simulink model "cv_model_CMORPH_5M"  (R2024a)
settings: Solver=ode23t  StartTime=0  StopTime=1431  FixedStep=0.0005  MaxStep=.01  RelTol=1e-4
model workspace (MAT data in the model file):
  test = 0
undefined symbols (not defined in the file): A_cheb_09_1, B_cheb_09_1, C_cheb_09_1
libraries: simulink_extras x2, SignalEditorBlockLib x1
(part 2 of 3)

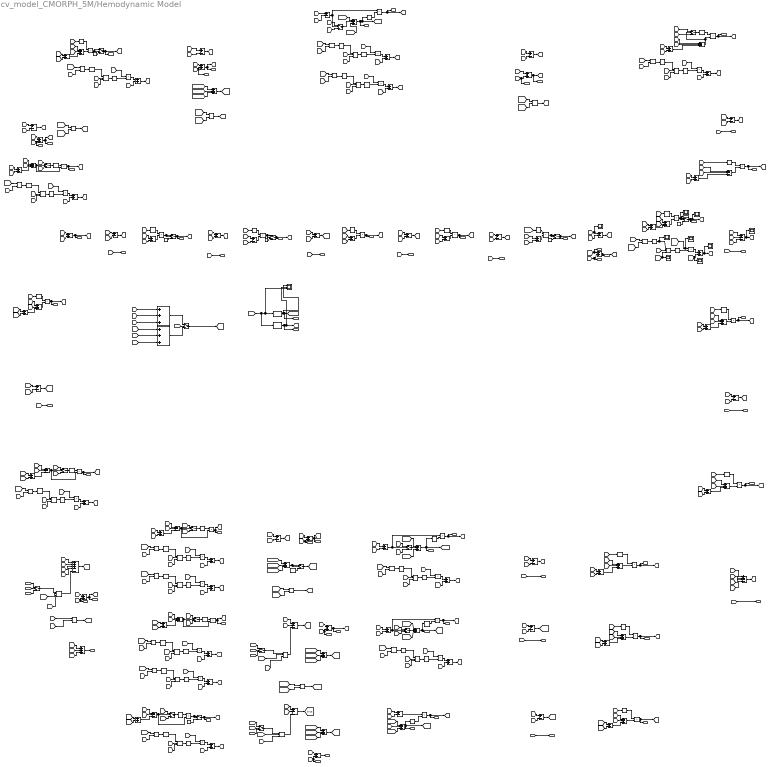
== system cv_model_CMORPH_5M/Hemodynamic Model ==
  note: Zero Pressure Volume
  note: Zero Pressure Volume
  note: Zero Pressure Volume
  note: Reduced Compliance at Negative Pressure
  note: Reduced Compliance at Negative Pressure
  note: Zero Pressure Volume
  note: Total Volume
  note: Zero Pressure Volume
  note: Update Zero Pressure Volume from Reflex
  note: Zero Pressure Volume
  note: Update Zero Pressure Volume from Reflex
  note: Zero Pressure Volume
  note: Zero Pressure Volume
  note: Zero Pressure Volume
  note: Zero Pressure Volume
  note: Zero Pressure Volume
  note: Total Volume
  note: Update Zero Pressure Volume from Reflex
  note: Total Volume
  note: Flow into Right Atrium
  note: Flow into Compartment 14
  note: Flow Out of Compartment 9
  note: Total Volume
  note: Vessel Collapse Before
  note: Vessel Collapse After
  note: Flow Out of Compartment 11
  note: Total Volume
  note: Flow Out of Compartment 13
  note: Vessel Collapse
  note: Lower Body Microvascular Resistance
  note: Flow into Compartment 12
  note: Splanchnic Circulation Microvascular Resistance
  note: Vessel Collapse
  note: Flow into Compartment 10
  note: Renal Circulation Microvascular Resistance
  note: Vessel Collapse
  note: Flow into Compartment 8
  note: 2: Brachiocephalic Arteries
  note: Flow into Compartment 7
  note: Upper Body Microvascular Resistance
  note: Vessel Collapse After
  note: Flow into Compartment 3
  note: Vessel Collapse Model
  note: Flow into Compartment 2
  note: Vessel Collapse Before
  note: Flow into Compartment 6
  note: 3: Upper Body Arteries
  note: 6: Thoracic Aorta
  note: 7: Abdominal Aorta
  note: 8: Renal Arteries
  note: 9: Renal Veins
  note: 10: Splanchnic Arteries
  note: 11: Splanchnic Veins
  note: 12: Lower Body Arteries
  note: 13: Lower Body Veins
  note: Vessel Collapse Before
  note: Vessel Collapse After
  note: 14: Abdominal Veins
  note: Flow into Compartment 15
  note: Total Volume
  note: Vessel Collapse
  note: 15: Thoracic IVC
  note: Flow Out of Compartment 15
  note: 4: Upper Body Veins
  note: Vessel Collapse
  note: Flow into Compartment 5
  note: 5: SVC
  note: 1: Ascending Aorta
  note: Vessel Collapse
  note: Total Volume
  note: Flow Out of Compartment 5
  note: Right Atrium
  note: Flow into Right Ventricle
  note: Right Ventricle
  note: Flow into Pulmonary Arteries
  note: Pulmonary Arteries
  note: Pulmonary Microvascular Resistance
  note: Pulmonary Veins
  note: Flow Out of Pulmonary Veins
  note: Left Atrium
  note: Flow into Left Ventricle
  note: Left Ventricle
  note: Flow Out of Left Ventricle
  note: Vessel Collapse
  note: Total Volume
  note: Total Hydrostatic Pressure into lower venous system for interstitial flow division
  note: Interstitial Flow to Splanchnic Veins
  note: Interstitial Flow to Lower Body Veins
  note: Interstitial Flow to Abdominal Veins
  note: Transfer Function for Vint
  note: Transfer Function for Qint
  note: Flow and Volume to Interstitial Space
  note: Reduced Compliance at Negative Pressure
  note: Reduced Compliance at Negative Pressure
  note: Reduced Compliance at Negative Pressure
  note: Reduced Compliance at Negative Pressure
  note: Zero Pressure Volume
  note: Zero Pressure Volume
  note: Update Zero Pressure Volume from Reflex
  Constant{1..6} (6 alike) : Constant  Value=0
  Math Function{,1,4,9..12,15..16,19..21,24,29,34,37..38,41,44..49} (24 alike) : Math  Operator=reciprocal  SignedPower=on
  Math Function{2,5,7,13,17,22,25..26,30..31,35,39,42,50} (14 alike) : Math  SignedPower=on
  Math Function{3,6,8,14,18,23,27..28,32..33,36,40,43,51} (14 alike) : Math  Operator=log  SignedPower=on
  Product{,1,4,7,10..11,14..15,18..19,22,25,28,31,34,37,40,43} (18 alike) : Product  InputSameDT=on  SaturateOnIntegerOverflow=on  OutDataTypeStr=Inherit: Same as first input
  Product{2,5,8,12,16,20,23,26,29,32,35,38,41,44} (14 alike) : Product  Inputs=*/  InputSameDT=on  SaturateOnIntegerOverflow=on  OutDataTypeStr=Inherit: Same as first input
  Product{3,6,9,13,17,21,24,27,30,33,36,39,42,45} (14 alike) : Product  Inputs=**/  InputSameDT=on  SaturateOnIntegerOverflow=on  OutDataTypeStr=Inherit: Same as first input
  Scope : Scope  NumInputPorts=3
  Scope{1..9} (9 alike) : Scope
  Sum{,3,12,16,20,44..48,52,55..68} (25 alike) : Sum  Inputs=+-  InputSameDT=on  SaturateOnIntegerOverflow=on  OutDataTypeStr=Inherit: Same as first input
  Sum{1..2,21,23,28,33,36,49,54,70..71} (11 alike) : Sum  Inputs=+--  InputSameDT=on  SaturateOnIntegerOverflow=on  OutDataTypeStr=Inherit: Same as first input
  Sum{9..11,13,17,37,40} (7 alike) : Sum  Inputs=+-+  InputSameDT=on  SaturateOnIntegerOverflow=on  OutDataTypeStr=Inherit: Same as first input
  Sum{4..6,8,14,18,24..27,29..31,34..35,38..39,41..43,50..51,77..92} (38 alike) : Sum  InputSameDT=on  SaturateOnIntegerOverflow=on  OutDataTypeStr=Inherit: Same as first input
  Sum{7,15,19,22,32,69,73..76,93} (11 alike) : Sum  Inputs=+++  InputSameDT=on  SaturateOnIntegerOverflow=on  OutDataTypeStr=Inherit: Same as first input
  Sum53 : Sum  Inputs=+---  InputSameDT=on  SaturateOnIntegerOverflow=on  OutDataTypeStr=Inherit: Same as first input
  Sum72 : Sum  Inputs=+++--  InputSameDT=on  SaturateOnIntegerOverflow=on  OutDataTypeStr=Inherit: Same as first input
  Switch{1..14,21} (15 alike) : Switch
  Switch{16,18..20} (4 alike) : Switch  Threshold=0.5
  Switch17 : Switch  Criteria=u2 > Threshold  Threshold=5
  Transfer Fcn (with initial states) : simulink_extras/Additional Linear/Transfer Fcn (with initial states)  N=[1 0]  D=[276 1]  X0=0
  Transfer Fcn (with initial states)1 : simulink_extras/Additional Linear/Transfer Fcn (with initial states)  N=[1]  D=[276 1]  X0=0
  ZV1 : Constant  Value=5
  kool{1..20} (20 alike) : Product  Inputs=**  InputSameDT=on  SaturateOnIntegerOverflow=on  OutDataTypeStr=Inherit: Same as first input
  kool21 : Product  Inputs=*/*  InputSameDT=on  SaturateOnIntegerOverflow=on  OutDataTypeStr=Inherit: Same as first input
  kool22 : Product  Inputs=*/*  InputSameDT=on  SaturateOnIntegerOverflow=on  OutDataTypeStr=Inherit: Same as first input
  kool23 : Product  Inputs=*/*  InputSameDT=on  SaturateOnIntegerOverflow=on  OutDataTypeStr=Inherit: Same as first input
  kool{24..29} (6 alike) : Product  Inputs=*/  InputSameDT=on  SaturateOnIntegerOverflow=on  OutDataTypeStr=Inherit: Same as first input
  Qlo : Outport
  Q2i : Outport  Port=2
  Q3i : Outport  Port=3
  Q4i : Outport  Port=4
  Q5i : Outport  Port=5
  Q5o : Outport  Port=6
  Q6i : Outport  Port=7
  Q7i : Outport  Port=8
  Q8i : Outport  Port=9
  Q9i : Outport  Port=10
  Q9o : Outport  Port=11
  Q10i : Outport  Port=12
  Q11i : Outport  Port=13
  Q11o : Outport  Port=14
  Q12i : Outport  Port=15
  Q13i : Outport  Port=16
  Q13o : Outport  Port=17
  Q14i : Outport  Port=18
  Q15i : Outport  Port=19
  Q15o : Outport  Port=20
  Qrai : Outport  Port=21
  Qri : Outport  Port=22
  Qro : Outport  Port=23
  Qpv : Outport  Port=24
  Qlai : Outport  Port=25
  Qli : Outport  Port=26
  Qint : Outport  Port=27
  Vint : Outport  Port=28
  RubNew : Outport  Port=29
  RrcNew : Outport  Port=30
  RscNew : Outport  Port=31
  RlcNew : Outport  Port=32
  zv1 : Outport  Port=33
  zv2 : Outport  Port=34
  zv3 : Outport  Port=35
  zv4 : Outport  Port=36
  zv5 : Outport  Port=37
  zv6 : Outport  Port=38
  zv7 : Outport  Port=39
  zv8 : Outport  Port=40
  zv9 : Outport  Port=41
  zv10 : Outport  Port=42
  zv11 : Outport  Port=43
  zv12 : Outport  Port=44
  zv13 : Outport  Port=45
  zv14 : Outport  Port=46
  zv15 : Outport  Port=47
  zvra : Outport  Port=48
  zvrv : Outport  Port=49
  zvpa : Outport  Port=50
  zvpv : Outport  Port=51
  zvla : Outport  Port=52
  zvlv : Outport  Port=53
  V3a : Outport  Port=54
  V4a : Outport  Port=55
  V5a : Outport  Port=56
  V9a : Outport  Port=57
  V11a : Outport  Port=58
  V13a : Outport  Port=59
  V14a : Outport  Port=60
  Vlva : Outport  Port=61
  Vl_dist : Outport  Port=62
  Qlo1 : Outport  Port=63
  tag scope: C11neg=global, C14neg=global, C3neg=global, C4neg=global, C5neg=global, C9neg=global, Q10i=global, Q11i=global, Q11o=global, Q12i=global, Q13i=global, Q13o=global, Q15i=global, Q15o=global, Q2i=global, Q3i=global, Q4i=global, Q5i=global, Q5o=global, Q6i=global, Q7i=global, Q8i=global, Q9i=global, Q9o=global, Qint=global, Qlai=global, Qli=global, Qlo=global, Qpv=global, Qrai=global, Qri=global, Qro=global, R11a=global, R11b=global, R13b=global, R14a=global, R1a=global, R3b=global, R4a=global, R5a=global, R9a=global, R9b=global, RlcNew=global, RrcNew=global, Rrcb=global, RscNew=global, Rscb=global, RubNew=global, Ruba=global, Rubb=global, V11a=global, V14a=global, V3a=global, V4a=global, V5a=global, V9a=global, Vint=global, Vl=global, ZV11=global, ZV13=global, ZV4=global, ZV9=global, dV10=global, dV11=global, dV12=global, dV13=global, dV14=global, dV15=global, dV1=global, dV2=global, dV3=global, dV4=global, dV5=global, dV6=global, dV7=global, dV8=global, dV9=global, dVl=global, dVla=global, dVpa=global, dVpv=global, dVr=global, dVra=global, hTotal=global
  wires:
  [P1] -> Sum1/1
  Sum1/1 -> kool4/2
  kool4/1 -> Q2i/1, [Q2i]
  Math Function/1 -> kool4/1
  [R2] -> Math Function/1
  [P2] -> Sum1/2
  Sum78/1 -> Sum1/3
  [R3b] -> Switch3/3
  Sum4/1 -> [R3b]
  [P3] -> Sum2/2
  [ZV3] -> Product3/3
  [P2] -> Sum2/1
  Math Function2/1 -> Product1/2
  Math Function3/1 -> Product3/1
  Product1/1 -> Sum4/1
  [V3a] -> Product3/2
  Product2/1 -> Math Function3/1
  [Rhigh] -> Product1/1
  Sum2/1 -> kool1/2, Switch3/2
  kool1/1 -> [Q3i], Q3i/1
  [R3] -> Switch3/1
  Product3/1 -> Math Function2/1
  [epsilon] -> Product2/1
  Sum79/1 -> Sum2/3
  Math Function1/1 -> kool1/1
  Switch3/1 -> Math Function1/1
  [R3] -> Sum4/2
  [Rhigh] -> Product2/2
  Sum8/1 -> [Rubb]
  Math Function4/1 -> Product/2
  Math Function7/1 -> Product7/2
  Product8/1 -> Math Function8/1
  Product9/1 -> Math Function7/1
  Math Function6/1 -> Product6/1
  [V4a] -> Product9/2
  [ZV3] -> Product6/3
  [P4] -> Sum3/2
  Product7/1 -> Sum8/1
  Product4/1 -> Sum6/1
  Sum3/1 -> Product/1, Switch1/2
  [epsilon] -> Product8/1
  [ZV4] -> Product9/3
  [Rhigh] -> Product7/1
  [Rub] -> Sum8/2
  Math Function8/1 -> Product9/1
  [Rhigh] -> Product5/2
  [Rhigh] -> Product8/2
  [rupdelt] -> Sum7/1
  Math Function5/1 -> Product4/2
  Sum5/1 -> [V3a], V3a/1
  [Rubb] -> Switch1/3
  Product5/1 -> Math Function6/1
  [ZV3] -> zv3/1, Sum5/2
  [Ruba] -> Switch1/1
  [V3] -> Sum5/1
  [V3a] -> Product6/2
  Product6/1 -> Math Function5/1
  [epsilon] -> Product5/1
  Switch1/1 -> Sum7/2
  [Rub] -> Sum6/2
  [rupdeltCP] -> Sum7/3
  Sum6/1 -> [Ruba]
  [Rhigh] -> Product4/1
  Sum7/1 -> [RubNew], Math Function4/1, RubNew/1
  [P3] -> Sum3/1
  Product/1 -> [Q4i], Q4i/1
  [P6] -> Sum9/2
  [P1] -> Sum9/1
  [R6] -> Math Function9/1
  Sum82/1 -> Sum9/3
  Sum9/1 -> kool2/2
  kool2/1 -> [Q6i], Q6i/1
  Math Function9/1 -> kool2/1
  Sum83/1 -> Sum10/3
  Math Function10/1 -> kool3/1
  kool3/1 -> [Q7i], Q7i/1
  [R7] -> Math Function10/1
  Sum10/1 -> kool3/2
  [P7] -> Sum10/2
  [P6] -> Sum10/1
  [P8] -> Sum11/2
  [R8] -> Math Function11/1
  Sum11/1 -> kool5/2
  [P7] -> Sum11/1
  Sum85/1 -> Sum11/3
  kool5/1 -> [Q8i], Q8i/1
  Math Function11/1 -> kool5/1
  [Rrcb] -> Switch2/3
  [Rhigh] -> Product11/1
  Sum14/1 -> [Rrcb]
  Product10/1 -> Q9i/1, [Q9i]
  Math Function13/1 -> Product11/2
  Switch2/1 -> Sum15/2
  [P9] -> Sum12/2
  [epsilon] -> Product12/1
  [V9a] -> Product13/2
  Product13/1 -> Math Function13/1
  Math Function12/1 -> Product10/2
  [P8] -> Sum12/1
  [Rhigh] -> Product12/2
  Product12/1 -> Math Function14/1
  [rkdeltCP] -> Sum15/3
  [ZV9] -> Product13/3
  Product11/1 -> Sum14/1
  [Rrc] -> Switch2/1
  [Rrc] -> Sum14/2
  Sum12/1 -> Product10/1, Switch2/2
  [rkdelt] -> Sum15/1
  Sum15/1 -> RrcNew/1, [RrcNew], Math Function12/1
  Math Function14/1 -> Product13/1
  [P10] -> Sum13/2
  [R10] -> Math Function15/1
  Math Function15/1 -> kool6/1
  Sum87/1 -> Sum13/3
  kool6/1 -> [Q10i], Q10i/1
  [P7] -> Sum13/1
  Sum13/1 -> kool6/2
  [Rscb] -> Switch4/3
  [P11] -> Sum16/2
  [ZV11] -> Product17/3
  [epsilon] -> Product16/1
  Math Function17/1 -> Product15/2
  [Rsc] -> Switch4/1
  Product15/1 -> Sum18/1
  [rspdelt] -> Sum19/1
  Product16/1 -> Math Function18/1
  Math Function18/1 -> Product17/1
  Product17/1 -> Math Function17/1
  [V11a] -> Product17/2
  [rspdeltCP] -> Sum19/3
  Switch4/1 -> Sum19/2
  [Rhigh] -> Product16/2
  Sum18/1 -> [Rscb]
  [Rhigh] -> Product15/1
  Math Function16/1 -> Product14/2
  Sum16/1 -> Product14/1, Switch4/2
  Sum19/1 -> [RscNew], Math Function16/1, RscNew/1
  Product14/1 -> Q11i/1, [Q11i]
  [P10] -> Sum16/1
  [Rsc] -> Sum18/2
  [P12] -> Sum17/2
  Sum89/1 -> Sum17/3
  Math Function19/1 -> kool7/1
  Sum17/1 -> kool7/2
  [R12] -> Math Function19/1
  [P7] -> Sum17/1
  kool7/1 -> [Q12i], Q12i/1
  Math Function20/1 -> Product18/2
  Sum22/1 -> [RlcNew], Math Function20/1, RlcNew/1
  [rlldeltCP] -> Sum22/3
  [Rlc] -> Sum22/2
  Product18/1 -> Q13i/1, [Q13i]
  [rlldelt] -> Sum22/1
  [P13] -> Sum20/2
  Sum20/1 -> Product18/1
  [P12] -> Sum20/1
  [R13] -> Sum24/2
  [R13] -> Switch6/1
  [R13b] -> Switch6/3
  Sum24/1 -> [R13b]
  Product19/1 -> Sum24/1
  [Rhigh] -> Product19/1
  Product20/1 -> Math Function23/1
  [Rhigh] -> Product20/2
  Math Function22/1 -> Product19/2
  Math Function23/1 -> Product21/1
  Constant1/1 -> Switch5/3
  [V14a] -> Product21/2
  [epsilon] -> Product20/1
  [ZV14] -> Product21/3
  kool8/1 -> Switch5/2, Switch5/1
  [P14] -> Sum21/2
  Switch5/1 -> [Q13o], Q13o/1
  Switch6/1 -> Math Function21/1
  Sum21/1 -> kool8/2, Switch6/2
  Sum90/1 -> Sum21/3
  Product21/1 -> Math Function22/1
  Math Function21/1 -> kool8/1
  [P13] -> Sum21/1
  [R11] -> Sum27/2
  [epsilon] -> Product26/1
  Product26/1 -> Math Function28/1
  Math Function25/1 -> Product25/2
  kool9/1 -> Q11o/1, [Q11o]
  [ZV14] -> Product27/3
  Product23/1 -> Math Function27/1
  Product27/1 -> Math Function25/1
  Math Function27/1 -> Product24/1
  [epsilon] -> Product23/1
  [V11] -> Sum26/1
  Math Function28/1 -> Product27/1
  [R11] -> Sum25/2
  [V14a] -> Product27/2
  [Rhigh] -> Product25/1
  Switch7/1 -> Math Function24/1
  [Rhigh] -> Product22/1
  [Rhigh] -> Product23/2
  Product24/1 -> Math Function26/1
  Product25/1 -> Sum25/1
  Product22/1 -> Sum27/1
  Sum25/1 -> [R11b]
  [P11] -> Sum23/1
  Sum23/1 -> Switch7/2, kool9/2
  Sum26/1 -> [V11a], V11a/1
  [R11a] -> Switch7/1
  Math Function26/1 -> Product22/2
  [ZV11] -> Product24/3
  [P14] -> Sum23/2
  [ZV11] -> zv11/1, Sum26/2
  Math Function24/1 -> kool9/1
  [R11b] -> Switch7/3
  [Rhigh] -> Product26/2
  [V11a] -> Product24/2
  Sum27/1 -> [R11a]
  Sum88/1 -> Sum23/3
  [Rhigh] -> Product31/1
  [R9] -> Sum29/2
  [V14a] -> Product33/2
  Switch8/1 -> Math Function29/1
  Product31/1 -> Sum29/1
  Math Function33/1 -> Product33/1
  Math Function32/1 -> Product30/1
  [Rhigh] -> Product32/2
  kool10/1 -> Q9o/1, [Q9o]
  [V9] -> Sum30/1
  Math Function30/1 -> Product31/2
  [epsilon] -> Product29/1
  [P14] -> Sum28/2
  [ZV9] -> zv9/1, Sum30/2
  [Rhigh] -> Product28/1
  Sum30/1 -> [V9a], V9a/1
  [Rhigh] -> Product29/2
  Math Function29/1 -> kool10/1
  [ZV14] -> Product33/3
  [P9] -> Sum28/1
  [epsilon] -> Product32/1
  Sum86/1 -> Sum28/3
  [R9a] -> Switch8/1
  Product29/1 -> Math Function32/1
  Product28/1 -> Sum31/1
  [R9b] -> Switch8/3
  Sum31/1 -> [R9a]
  [R9] -> Sum31/2
  Product32/1 -> Math Function33/1
  Math Function31/1 -> Product28/2
  [ZV9] -> Product30/3
  Sum28/1 -> kool10/2, Switch8/2
  Product33/1 -> Math Function30/1
  Product30/1 -> Math Function31/1
  [V9a] -> Product30/2
  Sum29/1 -> [R9b]
  [Q13o] -> Sum32/3
  Sum32/1 -> Q14i/1
  [Q11o] -> Sum32/2
  [Q9o] -> Sum32/1
  Math Function36/1 -> Product36/1
  [R14] -> Switch9/3
  [R14a] -> Switch9/1
  Switch9/1 -> Math Function34/1
  [ZV14] -> Sum34/2, zv14/1
  Sum35/1 -> [R14a]
  Math Function35/1 -> Product34/2
  [P15] -> Sum33/2
  [Rhigh] -> Product34/1
  [V14] -> Sum34/1
  [V14a] -> Product36/2
  Product35/1 -> Math Function36/1
  [R14] -> Sum35/2
  Sum91/1 -> Sum33/3
  [ZV14] -> Product36/3
  [Rhigh] -> Product35/2
  Product36/1 -> Math Function35/1
  kool11/1 -> Q15i/1, [Q15i]
  Math Function34/1 -> kool11/1
  [P14] -> Sum33/1
  Sum33/1 -> Switch9/2, kool11/2
  [epsilon] -> Product35/1
  Sum34/1 -> V14a/1, [V14a]
  Product34/1 -> Sum35/1
  Sum92/1 -> Sum36/3
  [R15] -> Math Function37/1
  [P15] -> Sum36/1
  Sum36/1 -> kool12/2
  kool12/1 -> Q15o/1, [Q15o]
  [Pra] -> Sum36/2
  Math Function37/1 -> kool12/1
  [V4a] -> Product39/2
  Sum39/1 -> [R4a]
  Math Function39/1 -> Product37/2
  Product37/1 -> Sum39/1
  [Rhigh] -> Product37/1
  [R4] -> Sum39/2
  Product39/1 -> Math Function39/1
  [P5] -> Sum37/2
  [Rhigh] -> Product38/2
  Product38/1 -> Math Function40/1
  Math Function40/1 -> Product39/1
  [V4] -> Sum38/1
  Switch10/1 -> Q5i/1, [Q5i]
  [ZV4] -> Product39/3
  kool13/1 -> Switch10/2, Switch10/1
  Sum80/1 -> Sum37/3
  Math Function38/1 -> kool13/1
  [P4] -> Sum37/1
  Sum37/1 -> kool13/2
  [R4a] -> Math Function38/1
  Constant2/1 -> Switch10/3
  [epsilon] -> Product38/1
  Sum38/1 -> V4a/1, [V4a]
  Math Function42/1 -> Product40/2
  kool14/1 -> Q5o/1, [Q5o]
  [ZV5] -> zv5/1, Sum41/2
  Sum41/1 -> V5a/1, [V5a]
  [epsilon] -> Product41/1
  Math Function41/1 -> kool14/1
  [Rhigh] -> Product40/1
  Sum40/1 -> kool14/2, Switch11/2
  [P5] -> Sum40/1
  Math Function43/1 -> Product42/1
  [R5a] -> Switch11/1
  [ZV5] -> Product42/3
  [Pra] -> Sum40/2
  [R5] -> Sum42/2
  Product40/1 -> Sum42/1
  [V5] -> Sum41/1
  [Rhigh] -> Product41/2
  [V5a] -> Product42/2
  Product42/1 -> Math Function42/1
  Switch11/1 -> Math Function41/1
  [R5] -> Switch11/3
  Sum42/1 -> [R5a]
  Product41/1 -> Math Function43/1
  Sum81/1 -> Sum40/3
  [Q15o] -> Sum43/2
  [Q5o] -> Sum43/1
  Sum43/1 -> Qrai/1, [Qrai]
  [R_tri] -> Math Function44/1
  Sum44/1 -> kool15/2
  kool15/1 -> Switch12/1, Switch12/2
  Math Function44/1 -> kool15/1
  Constant3/1 -> Switch12/3
  [Pra] -> Sum44/1
  [Pr] -> Sum44/2
  Switch12/1 -> Qri/1, [Qri]
  [Ppa] -> Sum45/2
  kool16/1 -> Switch13/2, Switch13/1
  [Rpa] -> Math Function45/1
  Math Function45/1 -> kool16/1
  Constant4/1 -> Switch13/3
  Sum45/1 -> kool16/2
  Switch13/1 -> [Qro], Qro/1
  [Pr] -> Sum45/1
  [Ppv] -> Sum46/2
  [Ppa] -> Sum46/1
  kool17/1 -> [Qpv], Qpv/1
  Sum46/1 -> kool17/2
  [Rpc] -> Math Function46/1
  Math Function46/1 -> kool17/1
  [Rpv] -> Math Function47/1
  Sum47/1 -> kool18/2
  kool18/1 -> [Qlai], Qlai/1
  Math Function47/1 -> kool18/1
  [Ppv] -> Sum47/1
  [Pla] -> Sum47/2
  [Pla] -> Sum48/1
  [R_mitral] -> Math Function48/1
  Switch14/1 -> [Qli], Qli/1
  Math Function48/1 -> kool19/1
  kool19/1 -> Switch14/2, Switch14/1
  Constant5/1 -> Switch14/3
  Sum48/1 -> kool19/2
  [Pl] -> Sum48/2
  Product44/1 -> Math Function51/1
  [Rhigh] -> Product44/2
  Product45/1 -> Math Function50/1
  [R1a] -> Math Function49/1
  [ZVlv] -> zvlv/1, Sum50/2
  Math Function51/1 -> Scope9/1, Product45/1
  Math Function50/1 -> Product43/2
  [ZVlv] -> Scope8/1, Product45/3
  Sum51/1 -> Scope5/1, [R1a]
  [epsilon] -> Product44/1
  kool20/1 -> Switch21/1, Qlo1/1, Switch21/2, Scope2/1
  [P1] -> Sum49/2
  Sum49/1 -> kool20/2
  Math Function49/1 -> kool20/1
  [Rhigh] -> Scope7/1, Product43/1
  [Pl] -> Sum49/1
  [Vl_dist] -> Vl_dist/1, Sum50/1
  Sum50/1 -> [Vl], Vlva/1
  Product43/1 -> Sum51/1
  [R1] -> Scope6/1, Sum51/2
  [Vl] -> Product45/2
  Sum52/1 -> [dV6]
  [Q7i] -> Sum52/2
  [Q6i] -> Sum52/1
  [Q8i] -> Sum53/2
  Sum53/1 -> [dV7]
  [Q7i] -> Sum53/1
  [Q10i] -> Sum53/3
  [Q12i] -> Sum53/4
  [Q2i] -> Sum54/2
  Sum54/1 -> Scope4/1, [dV1]
  [Qlo] -> Sum54/1
  [Q6i] -> Sum54/3
  [Q3i] -> Sum55/2
  [Q2i] -> Sum55/1
  Sum55/1 -> [dV2]
  [Q3i] -> Sum56/1
  Sum56/1 -> [dV3]
  [Q4i] -> Sum56/2
  Sum57/1 -> [dV4]
  [Q4i] -> Sum57/1
  [Q5i] -> Sum57/2
  [Q5o] -> Sum58/2
  [Q5i] -> Sum58/1
  Sum58/1 -> [dV5]
  Sum59/1 -> [dV15]
  [Q15o] -> Sum59/2
  [Q15i] -> Sum59/1
  [Q9i] -> Sum60/2
  [Q8i] -> Sum60/1
  Sum60/1 -> [dV8]
  Sum61/1 -> [dV10]
  [Q11i] -> Sum61/2
  [Q10i] -> Sum61/1
  [Q13i] -> Sum62/2
  Sum62/1 -> [dV12]
  [Q12i] -> Sum62/1
  [Qrai] -> Sum63/1
  [Qri] -> Sum63/2
  Sum63/1 -> [dVra]
  [Qri] -> Sum64/1
  [Qro] -> Sum64/2
  Sum64/1 -> [dVr]
  Sum65/1 -> [dVpa]
  [Qpv] -> Sum65/2
  [Qro] -> Sum65/1
  Sum/1 -> [dVpv]
  [Qpv] -> Sum/1
  [Qlai] -> Sum/2
  Sum66/1 -> [dVla]
  [Qlai] -> Sum66/1
  [Qli] -> Sum66/2
  [Qli] -> Scope3/1, Sum67/1
  Sum67/1 -> [dVl]
  [Qlo] -> Sum67/2
  [Q9i] -> Sum68/1
  Sum68/1 -> [dV9]
  [Q9o] -> Sum68/2
  [Qint] -> kool21/3
  [hTotal] -> kool21/2
  [Q11o] -> Sum70/2
  [Q11i] -> Sum70/1
  kool21/1 -> Sum70/3
  Sum71/1 -> [dV13]
  [hTotal] -> kool22/2
  [Qint] -> kool22/3
  [Q13i] -> Sum71/1
  [Q13o] -> Sum71/2
  Sum72/1 -> [dV14]
  kool23/1 -> Sum72/5
  [Q13o] -> Sum72/3
  [hTotal] -> kool23/2
  [Q9o] -> Sum72/1
  [Q15i] -> Sum72/4
  [Qint] -> kool23/3
  [Q11o] -> Sum72/2
  Transfer Fcn (with initial states)1/1 -> Vint/1, Scope/2, [Vint]
  kool25/1 -> [C9neg]
  kool24/1 -> [C4neg]
  [ZVnom9] -> kool25/1
  [Pcol] -> kool26/2
  [Pcol] -> kool27/2
  kool27/1 -> [C11neg]
  [ZV14] -> kool26/1
  kool26/1 -> [C14neg]
  [ZVnom4] -> kool24/1
  [ZVnom11] -> kool27/1
  [Pcol] -> kool25/2
  [Pcol] -> kool24/2
  Sum73/1 -> [ZV11]
  [vspvodeltCP] -> Sum73/3
  [vspvodelt] -> Sum73/2
  [ZVnom11] -> Sum73/1
  ZV1/1 -> Switch17/3
  Sum74/1 -> Switch17/1, Switch17/2
  Switch17/1 -> [ZV9]
  [vkvodeltCP] -> Sum74/3
  [ZVnom9] -> Sum74/1
  [vkvodelt] -> Sum74/2
  Sum75/1 -> [ZV4]
  [vupvodeltCP] -> Sum75/3
  [vupvodelt] -> Sum75/2
  [ZVnom4] -> Sum75/1
  [ZV1] -> zv1/1
  [ZV2] -> zv2/1
  [ZV4] -> Sum38/2, zv4/1
  [ZV6] -> zv6/1
  [ZV7] -> zv7/1
  [ZV8] -> zv8/1
  [ZV10] -> zv10/1
  [ZV12] -> zv12/1
  [ZV13] -> Sum84/2, zv13/1
  Sum84/1 -> V13a/1
  [V13] -> Sum84/1
  [ZV15] -> zv15/1
  [Pcol] -> kool28/2
  [ZV3] -> kool28/1
  kool28/1 -> [C3neg]
  [Pcol] -> kool29/2
  [ZV5] -> kool29/1
  kool29/1 -> [C5neg]
  [ZVra] -> zvra/1
  [ZVrv] -> zvrv/1
  [ZVpa] -> zvpa/1
  [ZVpv] -> zvpv/1
  [ZVla] -> zvla/1
  [ZVnom13] -> Sum76/1
  Sum76/1 -> [ZV13]
  [vllvodeltCP] -> Sum76/3
  [vllvodelt] -> Sum76/2
  [Psrc1] -> Sum77/1
  [Ph1] -> Sum77/2
  Sum77/1 -> Sum49/3
  [Ph2] -> Sum78/2
  [Psrc2] -> Sum78/1
  [Ph3] -> Sum79/2
  [Psrc3] -> Sum79/1
  [Ph4] -> Sum80/2
  [Psrc4] -> Sum80/1
  [Ph5] -> Sum81/2
  [Psrc5] -> Sum81/1
  [Ph6] -> Sum82/2
  [Psrc6] -> Sum82/1
  [Ph7] -> Sum83/2
  [Psrc7] -> Sum83/1
  [Ph8] -> Sum85/2
  [Psrc8] -> Sum85/1
  [Ph9] -> Sum86/2
  [Psrc9] -> Sum86/1
  [Ph10] -> Sum87/2
  [Psrc10] -> Sum87/1
  [Psrc11] -> Sum88/1
  [Ph11] -> Sum88/2
  [Psrc12] -> Sum89/1
  [Ph12] -> Sum89/2
  [Psrc13] -> Sum90/1
  [Ph13] -> Sum90/2
  [Psrc14] -> Sum91/1
  [Ph14] -> Sum91/2
  [Psrc15] -> Sum92/1
  [Ph15] -> Sum92/2
  Sum70/1 -> [dV11]
  [Vmax] -> Transfer Fcn (with initial states)1/1, Scope/3, Transfer Fcn (with initial states)/1
  Switch19/1 -> kool23/1
  Switch16/1 -> kool22/1
  Switch18/1 -> kool21/1
  kool22/1 -> Sum71/3
  Transfer Fcn (with initial states)/1 -> Scope/1, Qint/1, [Qint]
  [h13] -> Switch16/1
  [hsrc13] -> Switch16/3
  [Ctrl] -> Switch16/2
  [h11] -> Switch18/1
  [hsrc11] -> Switch18/3
  [Ctrl] -> Switch18/2
  [h14] -> Switch19/1
  [hsrc14] -> Switch19/3
  [Ctrl] -> Switch19/2
  [h11] -> Sum69/1
  [h13] -> Sum69/2
  [h14] -> Sum69/3
  [hsrc11] -> Sum93/1
  [hsrc13] -> Sum93/2
  [hsrc14] -> Sum93/3
  [Ctrl] -> Switch20/2
  Sum69/1 -> Switch20/1
  Sum93/1 -> Switch20/3
  Switch20/1 -> [hTotal]
  Constant6/1 -> Switch21/3
  Switch21/1 -> Qlo/1, Scope1/1, [Qlo]

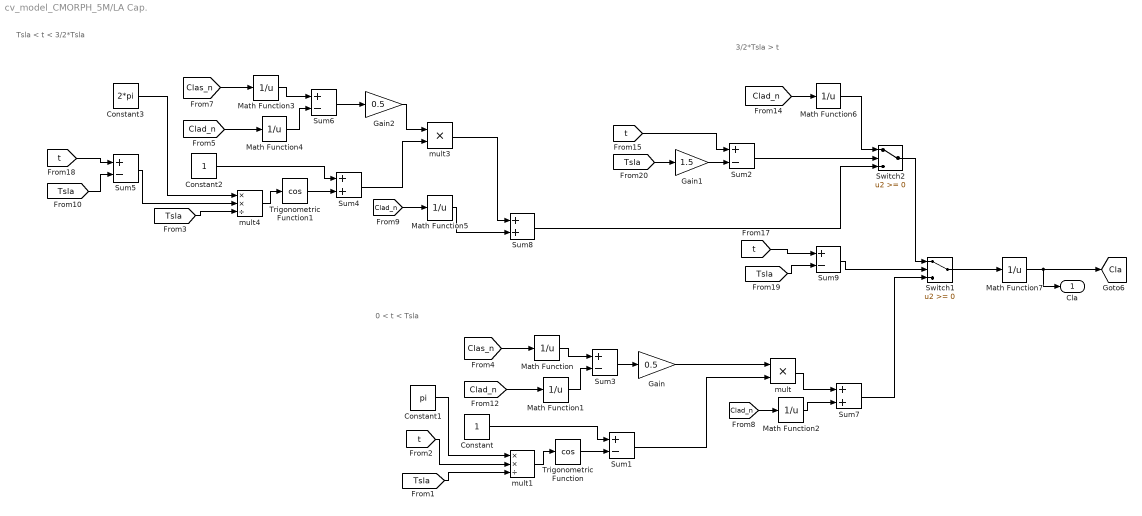
== system cv_model_CMORPH_5M/LA Cap. ==
  note: Tsla < t < 3/2*Tsla
  note: 3/2*Tsla > t
  note: 0 < t < Tsla
  Constant : Constant
  Constant1 : Constant  Value=pi
  Constant2 : Constant
  Constant3 : Constant  Value=2*pi
  Gain : Gain  Gain=0.5
  Gain1 : Gain  Gain=1.5
  Gain2 : Gain  Gain=0.5
  Math Function{,1..7} (8 alike) : Math  Operator=reciprocal  SignedPower=on
  Sum{1..3,5..6,9} (6 alike) : Sum  Inputs=+-  InputSameDT=on  SaturateOnIntegerOverflow=on  OutDataTypeStr=Inherit: Same as first input
  Sum4 : Sum  InputSameDT=on  SaturateOnIntegerOverflow=on  OutDataTypeStr=Inherit: Same as first input
  Sum7 : Sum  InputSameDT=on  SaturateOnIntegerOverflow=on  OutDataTypeStr=Inherit: Same as first input
  Sum8 : Sum  InputSameDT=on  SaturateOnIntegerOverflow=on  OutDataTypeStr=Inherit: Same as first input
  Switch1 : Switch
  Switch2 : Switch
  Trigonometric Function : Trigonometry  Operator=cos
  Trigonometric Function1 : Trigonometry  Operator=cos
  mult : Product  Inputs=**
  mult1 : Product  Inputs=**/
  mult3 : Product  Inputs=**
  mult4 : Product  Inputs=**/
  Cla : Outport
  tag scope: Cla=global
  wires:
  [Tsla] -> Sum9/2
  Sum9/1 -> Switch1/2
  [Clas_n] -> Math Function/1
  Sum3/1 -> Gain/1
  Gain/1 -> mult/1
  Constant/1 -> Sum1/1
  Trigonometric Function/1 -> Sum1/2
  Constant1/1 -> mult1/1
  mult1/1 -> Trigonometric Function/1
  [Tsla] -> mult1/3
  Sum1/1 -> mult/2
  [t] -> mult1/2
  mult/1 -> Sum7/1
  Math Function/1 -> Sum3/1
  [Clad_n] -> Math Function1/1
  Math Function1/1 -> Sum3/2
  [Clad_n] -> Math Function2/1
  Math Function2/1 -> Sum7/2
  Sum7/1 -> Switch1/3
  [t] -> Sum2/1
  [Tsla] -> Gain1/1
  Gain1/1 -> Sum2/2
  Switch2/1 -> Switch1/1
  Sum2/1 -> Switch2/2
  Sum6/1 -> Gain2/1
  Gain2/1 -> mult3/1
  Constant2/1 -> Sum4/1
  Trigonometric Function1/1 -> Sum4/2
  Constant3/1 -> mult4/1
  mult4/1 -> Trigonometric Function1/1
  [Tsla] -> mult4/3
  Sum4/1 -> mult3/2
  Sum5/1 -> mult4/2
  mult3/1 -> Sum8/1
  [Tsla] -> Sum5/2
  [Clas_n] -> Math Function3/1
  Math Function3/1 -> Sum6/1
  [Clad_n] -> Math Function4/1
  Math Function4/1 -> Sum6/2
  [Clad_n] -> Math Function5/1
  Math Function5/1 -> Sum8/2
  [t] -> Sum5/1
  [t] -> Sum9/1
  Sum8/1 -> Switch2/3
  [Clad_n] -> Math Function6/1
  Math Function6/1 -> Switch2/1
  Switch1/1 -> Math Function7/1
  Math Function7/1 -> [Cla], Cla/1

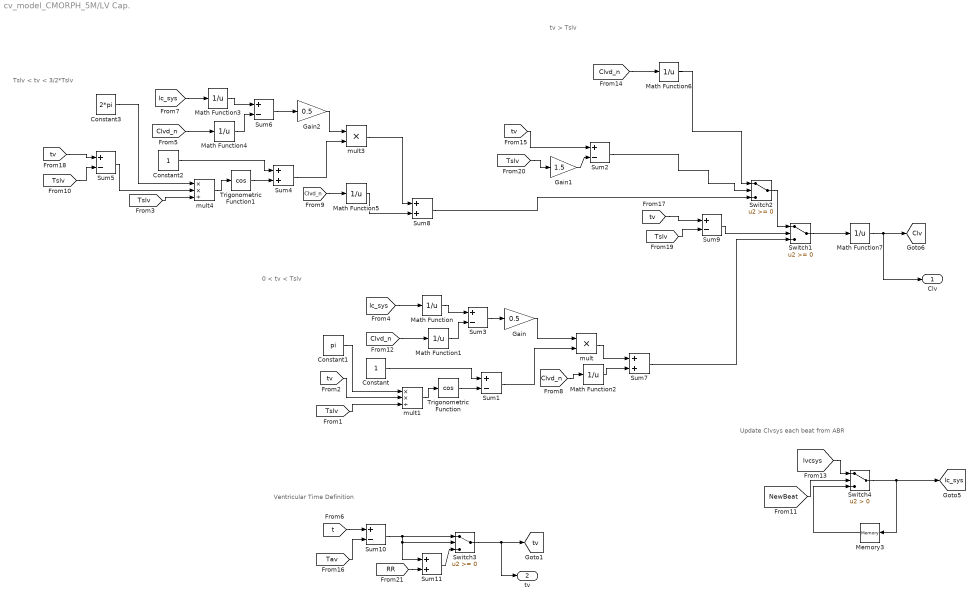
== system cv_model_CMORPH_5M/LV Cap. ==
  note: tv > Tslv
  note: Tslv < tv < 3/2*Tslv
  note: 0 < tv < Tslv
  note: Update Clvsys each beat from ABR
  note: Ventricular Time Definition
  Constant : Constant
  Constant1 : Constant  Value=pi
  Constant2 : Constant
  Constant3 : Constant  Value=2*pi
  Gain : Gain  Gain=0.5
  Gain1 : Gain  Gain=1.5
  Gain2 : Gain  Gain=0.5
  Math Function{,1..7} (8 alike) : Math  Operator=reciprocal  SignedPower=on
  Memory3 : Memory  InitialCondition=0.4  InheritSampleTime=on
  Sum{1..3,5..6,9..10} (7 alike) : Sum  Inputs=+-  InputSameDT=on  SaturateOnIntegerOverflow=on  OutDataTypeStr=Inherit: Same as first input
  Sum{4,7..8,11} (4 alike) : Sum  InputSameDT=on  SaturateOnIntegerOverflow=on  OutDataTypeStr=Inherit: Same as first input
  Switch1 : Switch
  Switch2 : Switch
  Switch3 : Switch
  Switch4 : Switch  Criteria=u2 > Threshold
  Trigonometric Function : Trigonometry  Operator=cos
  Trigonometric Function1 : Trigonometry  Operator=cos
  mult : Product  Inputs=**
  mult1 : Product  Inputs=**/
  mult3 : Product  Inputs=**
  mult4 : Product  Inputs=**/
  Clv : Outport
  tv : Outport  Port=2
  tag scope: Clv=global, lc_sys=global, tv=global
  wires:
  [Tslv] -> Sum9/2
  Sum9/1 -> Switch1/2
  [lc_sys] -> Math Function/1
  Sum3/1 -> Gain/1
  Gain/1 -> mult/1
  Constant/1 -> Sum1/1
  Trigonometric Function/1 -> Sum1/2
  Constant1/1 -> mult1/1
  mult1/1 -> Trigonometric Function/1
  [Tslv] -> mult1/3
  Sum1/1 -> mult/2
  [tv] -> mult1/2
  mult/1 -> Sum7/1
  Math Function/1 -> Sum3/1
  [Clvd_n] -> Math Function1/1
  Math Function1/1 -> Sum3/2
  [Clvd_n] -> Math Function2/1
  Math Function2/1 -> Sum7/2
  Sum7/1 -> Switch1/3
  [tv] -> Sum2/1
  [Tslv] -> Gain1/1
  Gain1/1 -> Sum2/2
  Switch2/1 -> Switch1/1
  Sum2/1 -> Switch2/2
  Sum6/1 -> Gain2/1
  Gain2/1 -> mult3/1
  Constant2/1 -> Sum4/1
  Trigonometric Function1/1 -> Sum4/2
  Constant3/1 -> mult4/1
  mult4/1 -> Trigonometric Function1/1
  [Tslv] -> mult4/3
  Sum4/1 -> mult3/2
  Sum5/1 -> mult4/2
  mult3/1 -> Sum8/1
  [Tslv] -> Sum5/2
  [lc_sys] -> Math Function3/1
  Math Function3/1 -> Sum6/1
  [Clvd_n] -> Math Function4/1
  Math Function4/1 -> Sum6/2
  [Clvd_n] -> Math Function5/1
  Math Function5/1 -> Sum8/2
  [tv] -> Sum5/1
  [tv] -> Sum9/1
  Sum8/1 -> Switch2/3
  [Clvd_n] -> Math Function6/1
  Math Function6/1 -> Switch2/1
  Switch1/1 -> Math Function7/1
  Math Function7/1 -> [Clv], Clv/1
  [NewBeat] -> Switch4/2
  Switch4/1 -> Memory3/1, [lc_sys]
  Memory3/1 -> Switch4/3
  [lvcsys] -> Switch4/1
  [t] -> Sum10/1
  [Tav] -> Sum10/2
  Sum10/1 -> Switch3/1, Switch3/2, Sum11/1
  Switch3/1 -> tv/1, [tv]
  [RR] -> Sum11/2
  Sum11/1 -> Switch3/3

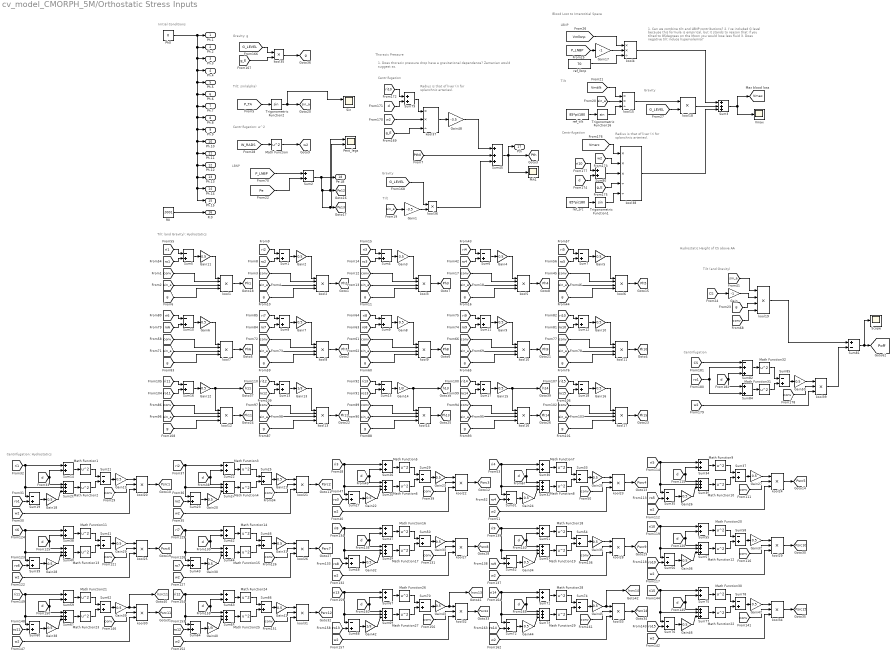
== system cv_model_CMORPH_5M/Orthostatic Stress Inputs ==
  note: Centrifugation
  note: Tilt (and Gravity)
  note: Gravity
  note: Tilt
  note: LBNP
  note: Centrifugation
  note: Radius is that of liver (ri for splanchnic arteries).
  note: Gravity
  note: Tilt
  note: Centrifugation: Hydrostatics
  note: 1. Can we combine tilt and LBNP contributions?
      | 2. I've included G level because this formula is empirical, but it stands to reason that if you tilted to 85degrees on the Moon you would lose less fluid
      | 3. Does negative tilt induce hypervolemia?
  note: Hydrostatic Height of CS above AA
  note: Blood Lost to Interstitial Space
  note: Tilt: sin(alpha)
  note: Tilt (and Gravity): Hydrostatics
  note: Initial Conditions
  note: LBNP
  note: Thoracic Pressure
  note: 1. Does thoracic pressure drop have a gravitational dependence? Zamanian would suggest so.
  note: Centrifugation: w^2
  note: Gravity: g
  note: Centrifugation
  note: Radius is that of liver (ri for splanchnic arteries).
  Gain : Gain  Gain=-1
  Gain1 : Gain  Gain=-3.5  SaturateOnIntegerOverflow=on  OutDataTypeStr=Inherit: Same as input  ParamDataTypeStr=Inherit: Same as input
  Gain{2..12,15..16,18..39,41,43..47,50} (42 alike) : Gain  Gain=0.5  SaturateOnIntegerOverflow=on  OutDataTypeStr=Inherit: Same as input  ParamDataTypeStr=Inherit: Same as input
  Gain{13..14,40,42} (4 alike) : Gain  Gain=1/3  SaturateOnIntegerOverflow=on  OutDataTypeStr=Inherit: Same as input  ParamDataTypeStr=Inherit: Same as input
  Gain17 : Gain  Gain=-1  SaturateOnIntegerOverflow=on  OutDataTypeStr=Inherit: Same as input  ParamDataTypeStr=Inherit: Same as input
  Gain48 : Gain  Gain=-3.5  SaturateOnIntegerOverflow=on  OutDataTypeStr=Inherit: Same as input  ParamDataTypeStr=Inherit: Same as input
  Math Function{,1..32} (33 alike) : Math  Operator=square
  Pext_legs : Scope  NumInputPorts=2
  Ph0 : Constant  Value=0
  Pth1 : Scope
  R0 : Constant  Value=.0001
  Scope : Scope
  Sin : Scope  NumInputPorts=2
  Sum{1,4..13,15..19,21,23,25,27,29,31,33,35,37,39,41,43,46,48,50,52,54,56,58,60,62,64,66,68,70,72,74,76,78,85} (46 alike) : Sum  Inputs=-+  InputSameDT=on  SaturateOnIntegerOverflow=on  OutDataTypeStr=Inherit: Same as first input
  Sum{2,14,22,26,30,34,38,42,47,51,55,59,63,67,71,75,79..80,84} (19 alike) : Sum  InputSameDT=on  SaturateOnIntegerOverflow=on  OutDataTypeStr=Inherit: Same as first input
  Sum{3,20,24,28,32,36,40,44..45,49,53,57,61,65,69,73,77} (17 alike) : Sum  Inputs=+++  InputSameDT=on  SaturateOnIntegerOverflow=on  OutDataTypeStr=Inherit: Same as first input
  Sum81 : Sum  Inputs=+-  InputSameDT=on  SaturateOnIntegerOverflow=on  OutDataTypeStr=Inherit: Same as first input
  Sum82 : Sum  Inputs=-++  InputSameDT=on  SaturateOnIntegerOverflow=on  OutDataTypeStr=Inherit: Same as first input
  Trigonometric Function1 : Trigonometry
  Trigonometric Function16 : Trigonometry
  Trigonometric Function2 : Trigonometry
  Vmax : Scope
  kool{1..3,5..14,16..17,19} (16 alike) : Product  Inputs=****  InputSameDT=on  SaturateOnIntegerOverflow=on  OutDataTypeStr=Inherit: Same as first input
  kool15 : Product  Inputs=**/  InputSameDT=on  SaturateOnIntegerOverflow=on  OutDataTypeStr=Inherit: Same as first input
  kool18 : Product  Inputs=**  InputSameDT=on  SaturateOnIntegerOverflow=on  OutDataTypeStr=Inherit: Same as first input
  kool{20..34,39} (16 alike) : Product  Inputs=3  InputSameDT=on  SaturateOnIntegerOverflow=on  OutDataTypeStr=Inherit: Same as first input
  kool35 : Product  Inputs=**  InputSameDT=on  SaturateOnIntegerOverflow=on  OutDataTypeStr=Inherit: Same as first input
  kool36 : Product  Inputs=**  InputSameDT=on  SaturateOnIntegerOverflow=on  OutDataTypeStr=Inherit: Same as first input
  kool37 : Product  Inputs=**/  InputSameDT=on  SaturateOnIntegerOverflow=on  OutDataTypeStr=Inherit: Same as first input
  kool38 : Product  Inputs=***//  InputSameDT=on  SaturateOnIntegerOverflow=on  OutDataTypeStr=Inherit: Same as first input
  kool4 : Product  Inputs=**/  InputSameDT=on  SaturateOnIntegerOverflow=on  OutDataTypeStr=Inherit: Same as first input
  ref_lbnp : Constant  Value=70
  ref_src : Constant  Value=85*pi/180
  ref_tilt : Constant  Value=85*pi/180
  Ph.1 : Outport
  Ph.2 : Outport  Port=2
  Ph.3 : Outport  Port=3
  Ph.4 : Outport  Port=4
  Ph.5 : Outport  Port=5
  Ph.6 : Outport  Port=6
  Ph.7 : Outport  Port=7
  Ph.8 : Outport  Port=8
  Ph.9 : Outport  Port=9
  Ph.10 : Outport  Port=10
  Ph.11 : Outport  Port=11
  Ph.12 : Outport  Port=12
  Ph.13 : Outport  Port=13
  Ph.14 : Outport  Port=14
  Ph.15 : Outport  Port=15
  R.0 : Outport  Port=16
  Pth : Outport  Port=17
  Pe.LB : Outport  Port=18
  tag scope: Pe12=global, Pe13=global, Ph10=global, Ph11=global, Ph12=global, Ph13=global, Ph14=global, Ph15=global, Ph1=global, Ph2=global, Ph3=global, Ph4=global, Ph5=global, Ph6=global, Ph7=global, Ph8=global, Ph9=global, Poff=global, Psrc10=global, Psrc11=global, Psrc12=global, Psrc13=global, Psrc14=global, Psrc15=global, Psrc1=global, Psrc2=global, Psrc3=global, Psrc4=global, Psrc5=global, Psrc6=global, Psrc7=global, Psrc8=global, Psrc9=global, Pth=global, Vmax=global, g=global, h11=global, h13=global, h14=global, hsrc11=global, hsrc13=global, hsrc14=global, sin_a=global, w2=global
  wires:
  Ph0/1 -> Ph.8/1, Ph.15/1, Ph.14/1, Ph.13/1, Ph.12/1, Ph.11/1, Ph.10/1, Ph.9/1, Ph.7/1, Ph.6/1, Ph.5/1, Ph.4/1, Ph.3/1, Ph.2/1, Ph.1/1
  R0/1 -> R.0/1
  ref_tilt/1 -> Trigonometric Function16/1
  [Vmtilt] -> kool15/1
  Trigonometric Function16/1 -> kool15/3
  [conv] -> kool1/2
  [sin_a] -> kool1/3
  [ri1] -> Sum5/1
  [sin_a] -> kool19/1
  [g] -> kool19/3
  Trigonometric Function2/1 -> Sin/1, [sin_a]
  Gain11/1 -> kool1/1
  Gain/1 -> kool19/2
  [conv] -> kool19/4
  [g] -> kool1/4
  [P_TA] -> Trigonometric Function2/1
  kool1/1 -> [Ph1]
  Sum5/1 -> Gain11/1
  [ro1] -> Sum5/2
  [g] -> kool2/4
  [ri2] -> Sum1/1
  kool2/1 -> [Ph2]
  [conv] -> kool2/2
  [sin_a] -> kool2/3
  Gain2/1 -> kool2/1
  [ro2] -> Sum1/2
  Sum1/1 -> Gain2/1
  Sum4/1 -> Gain3/1
  kool3/1 -> [Ph3]
  [ri3] -> Sum4/1
  [conv] -> kool3/2
  [sin_a] -> kool3/3
  Gain3/1 -> kool3/1
  [ro3] -> Sum4/2
  [g] -> kool3/4
  [g] -> kool5/4
  kool5/1 -> [Ph4]
  Gain4/1 -> kool5/1
  [ri4] -> Sum6/1
  [sin_a] -> kool5/3
  [ro4] -> Sum6/2
  Sum6/1 -> Gain4/1
  [conv] -> kool5/2
  [sin_a] -> kool6/3
  [ro5] -> Sum7/2
  [ri5] -> Sum7/1
  Gain5/1 -> kool6/1
  [conv] -> kool6/2
  kool6/1 -> [Ph5]
  Sum7/1 -> Gain5/1
  [g] -> kool6/4
  [conv] -> kool10/2
  [ri9] -> Sum11/1
  Gain9/1 -> kool10/1
  kool10/1 -> [Ph9]
  [ri10] -> Sum12/1
  [ro10] -> Sum12/2
  kool11/1 -> [Ph10]
  [g] -> kool10/4
  Sum10/1 -> Gain6/1
  [conv] -> kool11/2
  [ri6] -> Sum10/1
  [g] -> kool9/4
  Gain10/1 -> kool11/1
  [ro8] -> Sum9/2
  Sum11/1 -> Gain9/1
  [conv] -> kool9/2
  [sin_a] -> kool7/3
  kool9/1 -> [Ph8]
  [g] -> kool7/4
  Sum12/1 -> Gain10/1
  Gain8/1 -> kool9/1
  [ri8] -> Sum9/1
  [sin_a] -> kool9/3
  Sum9/1 -> Gain8/1
  kool7/1 -> [Ph6]
  [conv] -> kool7/2
  [sin_a] -> kool10/3
  [ro9] -> Sum11/2
  [g] -> kool11/4
  Gain6/1 -> kool7/1
  [ro6] -> Sum10/2
  Sum8/1 -> Gain7/1
  [sin_a] -> kool11/3
  kool8/1 -> [Ph7]
  [ri7] -> Sum8/1
  [conv] -> kool8/2
  [sin_a] -> kool8/3
  Gain7/1 -> kool8/1
  [ro7] -> Sum8/2
  [g] -> kool8/4
  [conv] -> kool16/2
  [ri14] -> Sum17/1
  Gain15/1 -> [h14], kool16/1
  kool16/1 -> [Ph14]
  [ri15] -> Sum18/1
  [ro15] -> Sum18/2
  kool17/1 -> [Ph15]
  [g] -> kool16/4
  Sum16/1 -> Gain12/1
  [conv] -> kool17/2
  [ri11] -> Sum16/1
  [g] -> kool14/4
  Gain16/1 -> kool17/1
  [ro13] -> Sum15/2
  Sum17/1 -> Gain15/1
  [conv] -> kool14/2
  [sin_a] -> kool12/3
  kool14/1 -> [Ph13]
  [g] -> kool12/4
  Sum18/1 -> Gain16/1
  Gain14/1 -> [h13], kool14/1
  [ri13] -> Sum15/1
  [sin_a] -> kool14/3
  Sum15/1 -> Gain14/1
  kool12/1 -> [Ph11]
  [conv] -> kool12/2
  [sin_a] -> kool16/3
  [ro14] -> Sum17/2
  [g] -> kool17/4
  Gain12/1 -> kool12/1, [h11]
  [ro11] -> Sum16/2
  Sum13/1 -> Gain13/1
  [sin_a] -> kool17/3
  kool13/1 -> [Ph12]
  [ri12] -> Sum13/1
  [conv] -> kool13/2
  [sin_a] -> kool13/3
  Gain13/1 -> kool13/1
  [ro12] -> Sum13/2
  [g] -> kool13/4
  [sin_a] -> Gain1/1
  [sin_a] -> kool15/2
  [P_LNBP] -> Sum2/1
  [Pe] -> Sum2/2
  [CS] -> Gain/1
  Gain17/1 -> kool4/2
  [Vmlbnp] -> kool4/1
  ref_lbnp/1 -> kool4/3
  Sum3/1 -> [Vmax], Vmax/1
  kool4/1 -> Sum3/1
  [P_LNBP] -> Gain17/1
  kool15/1 -> kool18/1
  [G_LEVEL] -> kool18/2
  kool18/1 -> Sum3/2
  Math Function/1 -> [w2]
  [W_RADS] -> Math Function/1
  kool20/1 -> [Psrc1]
  [ro1] -> Sum19/2
  Sum19/1 -> Gain18/1
  [ri1] -> Sum14/1, Sum19/1, Sum20/2
  [d] -> Sum20/1, Sum14/2
  Gain18/1 -> Sum20/3
  Sum14/1 -> Math Function1/1
  Sum20/1 -> Math Function2/1
  Math Function2/1 -> Sum21/2
  Math Function1/1 -> Sum21/1
  Sum21/1 -> Gain19/1
  Gain19/1 -> kool20/1
  [conv] -> kool20/2
  [w2] -> kool20/3
  [conv] -> kool21/2
  Sum23/1 -> Gain20/1
  [w2] -> kool21/3
  Sum25/1 -> Gain21/1
  Sum22/1 -> Math Function3/1
  Gain20/1 -> Sum24/3
  Math Function3/1 -> Sum25/1
  Sum24/1 -> Math Function4/1
  kool21/1 -> [Psrc2]
  [ri2] -> Sum22/1, Sum23/1, Sum24/2
  Gain21/1 -> kool21/1
  Math Function4/1 -> Sum25/2
  [ro2] -> Sum23/2
  [d] -> Sum24/1, Sum22/2
  Gain23/1 -> kool22/1
  [ri3] -> Sum26/1, Sum27/1, Sum28/2
  Gain22/1 -> Sum28/3
  Sum28/1 -> Math Function6/1
  Sum26/1 -> Math Function5/1
  Math Function5/1 -> Sum29/1
  Sum29/1 -> Gain23/1
  [d] -> Sum28/1, Sum26/2
  [conv] -> kool22/2
  Sum27/1 -> Gain22/1
  [w2] -> kool22/3
  kool22/1 -> [Psrc3]
  Math Function6/1 -> Sum29/2
  [ro3] -> Sum27/2
  Gain25/1 -> kool23/1
  [ri4] -> Sum30/1, Sum31/1, Sum32/2
  Gain24/1 -> Sum32/3
  Sum32/1 -> Math Function8/1
  Sum30/1 -> Math Function7/1
  Math Function7/1 -> Sum33/1
  Sum33/1 -> Gain25/1
  [d] -> Sum32/1, Sum30/2
  [conv] -> kool23/2
  Sum31/1 -> Gain24/1
  [w2] -> kool23/3
  kool23/1 -> [Psrc4]
  Math Function8/1 -> Sum33/2
  [ro4] -> Sum31/2
  Gain27/1 -> kool24/1
  [ri5] -> Sum34/1, Sum35/1, Sum36/2
  Gain26/1 -> Sum36/3
  Sum36/1 -> Math Function10/1
  Sum34/1 -> Math Function9/1
  Math Function9/1 -> Sum37/1
  Sum37/1 -> Gain27/1
  [d] -> Sum36/1, Sum34/2
  [conv] -> kool24/2
  Sum35/1 -> Gain26/1
  [w2] -> kool24/3
  kool24/1 -> [Psrc5]
  Math Function10/1 -> Sum37/2
  [ro5] -> Sum35/2
  [ro6] -> Sum39/2
  [conv] -> kool25/2
  Gain28/1 -> Sum40/3
  Sum39/1 -> Gain28/1
  [w2] -> kool25/3
  Sum41/1 -> Gain29/1
  Sum38/1 -> Math Function11/1
  Math Function11/1 -> Sum41/1
  Sum47/1 -> Math Function16/1
  [ri8] -> Sum47/1, Sum48/1, Sum49/2
  Sum49/1 -> Math Function17/1
  Math Function16/1 -> Sum50/1
  Sum50/1 -> Gain33/1
  Gain32/1 -> Sum49/3
  Gain33/1 -> kool27/1
  Math Function13/1 -> Sum41/2
  [conv] -> kool27/2
  [d] -> Sum49/1, Sum47/2
  Math Function17/1 -> Sum50/2
  [ro8] -> Sum48/2
  Sum48/1 -> Gain32/1
  kool29/1 -> [Psrc10]
  Math Function12/1 -> Sum58/2
  [ro10] -> Sum56/2
  [w2] -> kool29/3
  Math Function20/1 -> Sum58/1
  Sum57/1 -> Math Function12/1
  kool27/1 -> [Psrc8]
  Gain36/1 -> Sum57/3
  Sum56/1 -> Gain36/1
  [d] -> Sum57/1, Sum55/2
  kool25/1 -> [Psrc6]
  [d] -> Sum53/1, Sum51/2
  [conv] -> kool29/2
  kool28/1 -> [Psrc9]
  [conv] -> kool28/2
  Sum52/1 -> Gain34/1
  Gain34/1 -> Sum53/3
  Sum54/1 -> Gain35/1
  Sum51/1 -> Math Function18/1
  Gain35/1 -> kool28/1
  Gain37/1 -> kool29/1
  [w2] -> kool28/3
  [ri7] -> Sum42/1, Sum43/1, Sum44/2
  Math Function19/1 -> Sum54/2
  Gain30/1 -> Sum44/3
  Sum55/1 -> Math Function20/1
  Sum44/1 -> Math Function15/1
  Sum42/1 -> Math Function14/1
  Sum53/1 -> Math Function19/1
  Math Function14/1 -> Sum46/1
  Sum46/1 -> Gain31/1
  Math Function18/1 -> Sum54/1
  [w2] -> kool26/3
  kool26/1 -> [Psrc7]
  Sum43/1 -> Gain30/1
  [ri6] -> Sum38/1, Sum39/1, Sum40/2
  Gain31/1 -> kool26/1
  [d] -> Sum44/1, Sum42/2
  Math Function15/1 -> Sum46/2
  Sum58/1 -> Gain37/1
  [ri10] -> Sum55/1, Sum56/1, Sum57/2
  Sum40/1 -> Math Function13/1
  [ro7] -> Sum43/2
  Gain29/1 -> kool25/1
  [ro9] -> Sum52/2
  [d] -> Sum40/1, Sum38/2
  [ri9] -> Sum51/1, Sum52/1, Sum53/2
  [conv] -> kool26/2
  [w2] -> kool27/3
  [ro11] -> Sum60/2
  [conv] -> kool30/2
  Gain38/1 -> Sum61/3
  Sum60/1 -> Gain38/1
  [w2] -> kool30/3
  Sum62/1 -> Gain39/1
  Sum59/1 -> Math Function21/1
  Math Function21/1 -> Sum62/1
  Sum67/1 -> Math Function26/1
  [ri13] -> Sum67/1, Sum68/1, Sum69/2
  Sum69/1 -> Math Function27/1
  Math Function26/1 -> Sum70/1
  Sum70/1 -> Gain43/1
  Gain42/1 -> Sum69/3
  Gain43/1 -> [hsrc13], kool32/1
  Math Function23/1 -> Sum62/2
  [conv] -> kool32/2
  [d] -> Sum69/1, Sum67/2
  Math Function27/1 -> Sum70/2
  [ro13] -> Sum68/2
  Sum68/1 -> Gain42/1
  kool34/1 -> [Psrc15]
  Math Function22/1 -> Sum78/2
  [ro15] -> Sum76/2
  [w2] -> kool34/3
  Math Function30/1 -> Sum78/1
  Sum77/1 -> Math Function22/1
  kool32/1 -> [Psrc13]
  Gain46/1 -> Sum77/3
  Sum76/1 -> Gain46/1
  [d] -> Sum77/1, Sum75/2
  kool30/1 -> [Psrc11]
  [d] -> Sum73/1, Sum71/2
  [conv] -> kool34/2
  kool33/1 -> [Psrc14]
  [conv] -> kool33/2
  Sum72/1 -> Gain44/1
  Gain44/1 -> Sum73/3
  Sum74/1 -> Gain45/1
  Sum71/1 -> Math Function28/1
  Gain45/1 -> [hsrc14], kool33/1
  Gain47/1 -> kool34/1
  [w2] -> kool33/3
  [ri12] -> Sum63/1, Sum64/1, Sum65/2
  Math Function29/1 -> Sum74/2
  Gain40/1 -> Sum65/3
  Sum75/1 -> Math Function30/1
  Sum65/1 -> Math Function25/1
  Sum63/1 -> Math Function24/1
  Sum73/1 -> Math Function29/1
  Math Function24/1 -> Sum66/1
  Sum66/1 -> Gain41/1
  Math Function28/1 -> Sum74/1
  [w2] -> kool31/3
  kool31/1 -> [Psrc12]
  Sum64/1 -> Gain40/1
  [ri11] -> Sum59/1, Sum60/1, Sum61/2
  Gain41/1 -> kool31/1
  [d] -> Sum65/1, Sum63/2
  Math Function25/1 -> Sum66/2
  Sum78/1 -> Gain47/1
  [ri15] -> Sum75/1, Sum76/1, Sum77/2
  Sum61/1 -> Math Function23/1
  [ro12] -> Sum64/2
  Gain39/1 -> [hsrc11], kool30/1
  [ro14] -> Sum72/2
  [d] -> Sum61/1, Sum59/2
  [ri14] -> Sum71/1, Sum72/1, Sum73/2
  [conv] -> kool31/2
  [w2] -> kool32/3
  [G_LEVEL] -> kool35/1
  [g_E] -> kool35/2
  kool35/1 -> [g]
  Gain1/1 -> kool36/2
  [G_LEVEL] -> kool36/1
  [Pth0] -> Sum45/2
  kool36/1 -> Sum45/3
  Sum45/1 -> Pth1/1, [Pth], Pth/1
  [g_E] -> kool37/3
  [w2] -> kool37/2
  Sum79/1 -> kool37/1
  [ri10] -> Sum79/1
  [d] -> Sum79/2
  Gain48/1 -> Sum45/1
  kool37/1 -> Gain48/1
  [w2] -> kool38/2
  [Vmsrc] -> kool38/1
  ref_src/1 -> Trigonometric Function1/1
  Sum80/1 -> kool38/3
  [g_E] -> kool38/4
  Trigonometric Function1/1 -> kool38/5
  [ri10] -> Sum80/1
  [d] -> Sum80/2
  kool38/1 -> Sum3/3
  Sum81/1 -> Scope/1, [Poff]
  kool19/1 -> Sum81/1
  Sum84/1 -> Math Function31/1
  [ro1] -> Sum82/2, Sum84/2
  Sum85/1 -> Gain50/1
  Sum82/1 -> Math Function32/1
  Math Function31/1 -> Sum85/2
  Gain50/1 -> kool39/1
  [d] -> Sum84/1, Sum82/3
  [conv] -> kool39/2
  kool39/1 -> Sum81/2
  [w2] -> kool39/3
  Math Function32/1 -> Sum85/1
  [CS] -> Sum82/1
  Sum2/1 -> Pext_legs/2, [Pe13], Pext_legs/1, [Pe12], Pe.LB/1
